simulink model "sogi_pll"  (R2023b)
settings: Solver=VariableStepAuto  StartTime=0.0  StopTime=50e-2  RelTol=1e-3
libraries: spsAlphaBetaZerotodq0Lib x2
settings Model: Creator=sabar  LastModifiedBy=sabar

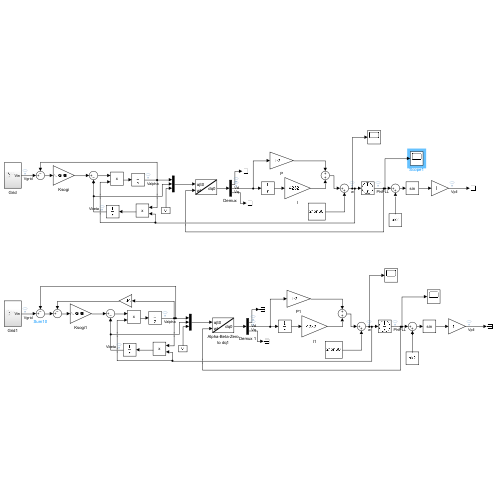
[thumbnail: Simulink's stored preview of the top-level diagram]
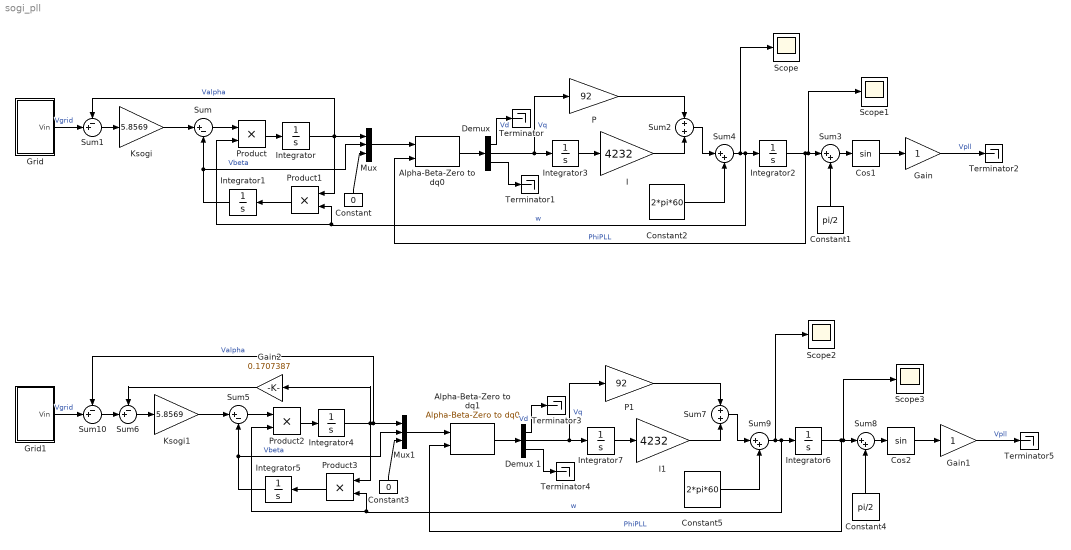
== system sogi_pll ==
  Alpha-Beta-Zero to dq0 : spsAlphaBetaZerotodq0Lib/Alpha-Beta-Zero to dq0  Alignment=Aligned with phase A axis
  Alpha-Beta-Zero to dq1 : spsAlphaBetaZerotodq0Lib/Alpha-Beta-Zero to dq0  Alignment=Aligned with phase A axis
  Constant : Constant  Value=0
  Constant1 : Constant  Value=pi/2
  Constant2 : Constant  Value=2*pi*60
  Constant3 : Constant  Value=0
  Constant4 : Constant  Value=pi/2
  Constant5 : Constant  Value=2*pi*60
  Cos1 : Trigonometry
  Cos2 : Trigonometry
  "Demux " : Demux  Outputs=3
  Demux 1 : Demux  Outputs=3
  Gain : Gain
  Gain1 : Gain
  Gain2 : Gain  Gain=0.1707387
  Grid : Subsystem
  Grid1 : Subsystem
  I : Gain  Gain=4232
  I1 : Gain  Gain=4232
  Integrator{,1,4..5} (4 alike) : Integrator  UpperSaturationLimit=1e3  LowerSaturationLimit=-1e3
  Integrator2 : Integrator  WrapState=on
  Integrator3 : Integrator
  Integrator6 : Integrator  WrapState=on
  Integrator7 : Integrator
  Ksogi : Gain  Gain=5.8569
  Ksogi1 : Gain  Gain=5.8569
  Mux : Mux  Inputs=3
  Mux1 : Mux  Inputs=3
  P : Gain  Gain=92
  P1 : Gain  Gain=92
  Product{,1..3} (4 alike) : Product
  Scope{,1..3} (4 alike) : Scope
  Sum : Sum  Inputs=|+-
  Sum1 : Sum  Inputs=-+|
  Sum10 : Sum  Inputs=-+|
  Sum2 : Sum  Inputs=+|+
  Sum{3..4,8..9} (4 alike) : Sum  Inputs=|++
  Sum5 : Sum  Inputs=|+-
  Sum6 : Sum  Inputs=-+|
  Sum7 : Sum  Inputs=+|+
  Terminator{,1..5} (6 alike) : Terminator
  wires:
  Sum2/1 -> Sum4/1
  Sum4/1 -> Scope/1, Product/2, Product1/2, Integrator2/1  "w"
  Constant/1 -> Mux/3
  Constant1/1 -> Sum3/2
  Sum3/1 -> Cos1/1
  Integrator2/1 -> Scope1/1, Sum3/1, Alpha-Beta-Zero to dq0/2  "PhiPLL"
  Cos1/1 -> Gain/1
  Gain/1 -> Terminator2/1  "Vpll"
  I/1 -> Sum2/2
  P/1 -> Sum2/1
  "Demux "/2 -> P/1, Integrator3/1  "Vq"
  Integrator3/1 -> I/1
  Constant2/1 -> Sum4/2
  "Demux "/3 -> Terminator1/1
  Integrator1/1 -> Mux/2, Sum/2  "Vbeta"
  "Demux "/1 -> Terminator/1  "Vd"
  Mux/1 -> Alpha-Beta-Zero to dq0/1
  Alpha-Beta-Zero to dq0/1 -> "Demux "/1
  Sum/1 -> Product/1
  Grid/1(Vin) -> Sum1/2  "Vgrid"
  Sum1/1 -> Ksogi/1
  Ksogi/1 -> Sum/1
  Product1/1 -> Integrator1/1
  Integrator/1 -> Product1/1, Mux/1, Sum1/1  "Valpha"
  Product/1 -> Integrator/1
  Product2/1 -> Integrator4/1
  Mux1/1 -> Alpha-Beta-Zero to dq1/1
  Ksogi1/1 -> Sum5/1
  Product3/1 -> Integrator5/1
  Sum5/1 -> Product2/1
  Demux 1/1 -> Terminator3/1  "Vd"
  Alpha-Beta-Zero to dq1/1 -> Demux 1/1
  Demux 1/3 -> Terminator4/1
  Constant5/1 -> Sum9/2
  P1/1 -> Sum7/1
  Cos2/1 -> Gain1/1
  Integrator7/1 -> I1/1
  Gain1/1 -> Terminator5/1  "Vpll"
  Integrator6/1 -> Scope3/1, Sum8/1, Alpha-Beta-Zero to dq1/2  "PhiPLL"
  Demux 1/2 -> P1/1, Integrator7/1  "Vq"
  I1/1 -> Sum7/2
  Sum7/1 -> Sum9/1
  Sum8/1 -> Cos2/1
  Integrator5/1 -> Mux1/2, Sum5/2  "Vbeta"
  Constant4/1 -> Sum8/2
  Constant3/1 -> Mux1/3
  Sum9/1 -> Scope2/1, Product2/2, Product3/2, Integrator6/1  "w"
  Sum6/1 -> Ksogi1/1
  Integrator4/1 -> Product3/1, Mux1/1, Sum10/1, Gain2/1  "Valpha"
  Gain2/1 -> Sum6/1
  Sum10/1 -> Sum6/2
  Grid1/1(Vin) -> Sum10/2  "Vgrid"

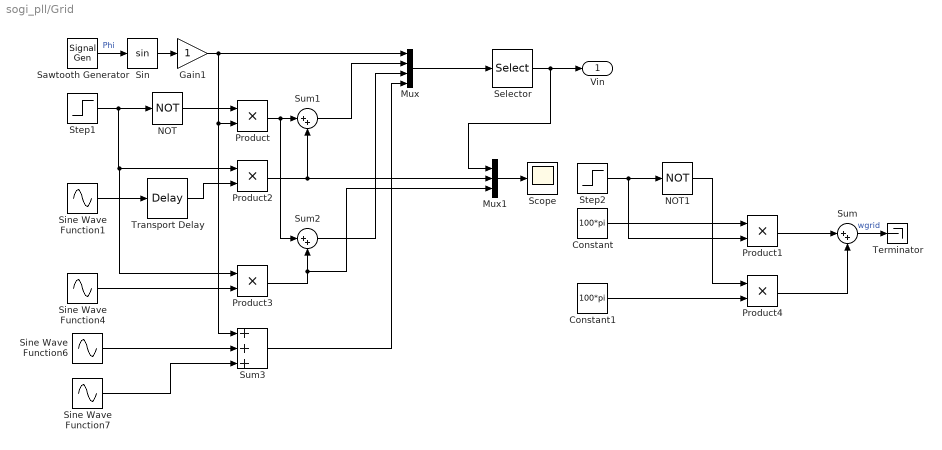
== system sogi_pll/Grid ==
  Constant : Constant  Value=100*pi
  Constant1 : Constant  Value=100*pi
  Gain1 : Gain
  Mux : Mux
  Mux1 : Mux  Inputs=3
  NOT : Logic  Operator=NOT  IconShape=distinctive  AllPortsSameDT=off  OutDataTypeStr=boolean
  NOT1 : Logic  Operator=NOT  IconShape=distinctive  AllPortsSameDT=off  OutDataTypeStr=boolean
  Product{,1..4} (5 alike) : Product
  Sawtooth Generator : SignalGenerator  WaveForm=sawtooth  Amplitude=pi  Frequency=314.159  Units=rad/sec
  Scope : Scope
  Selector : Selector  InputPortWidth=4  IndexOptions=Index vector (dialog)  Indices=1  OutputSizes=1
  Sin : Trigonometry
  Sine Wave Function1 : Sin  Frequency=314.159  SampleTime=0
  Sine Wave Function4 : Sin  Frequency=314.159  Phase=pi  SampleTime=0
  Sine Wave Function6 : Sin  Amplitude=1*0.1  Frequency=5*100*pi  SampleTime=0
  Sine Wave Function7 : Sin  Amplitude=1*0.05  Frequency=10*100*pi  SampleTime=0
  Step1 : Step  SampleTime=0
  Step2 : Step  Before=1  After=0  SampleTime=0
  Sum : Sum  Inputs=|++
  Sum1 : Sum  Inputs=|++
  Sum2 : Sum  Inputs=|++
  Sum3 : Sum  Inputs=+++
  Terminator : Terminator
  Transport Delay : TransportDelay  DelayTime=1000e-3
  Vin : Outport
  wires:
  Transport Delay/1 -> Product2/2
  Sine Wave Function7/1 -> Sum3/3
  Sum/1 -> Terminator/1  "wgrid"
  Sum3/1 -> Mux/4
  Constant/1 -> Product1/1
  Sine Wave Function1/1 -> Transport Delay/1
  Sin/1 -> Gain1/1
  Sum2/1 -> Mux/3
  Sawtooth Generator/1 -> Sin/1  "Phi"
  Product3/1 -> Mux1/3, Sum2/2
  Step2/1 -> Product1/2, NOT1/1
  Sine Wave Function4/1 -> Product3/2
  NOT1/1 -> Product4/1
  Sine Wave Function6/1 -> Sum3/2
  Mux/1 -> Selector/1
  Mux1/1 -> Scope/1
  NOT/1 -> Product/1
  Gain1/1 -> Sum3/1, Product/2, Mux/1
  Product2/1 -> Mux1/2, Sum1/2
  Product/1 -> Sum2/1, Sum1/1
  Step1/1 -> Product3/1, Product2/1, NOT/1
  Product1/1 -> Sum/1
  Sum1/1 -> Mux/2
  Selector/1 -> Mux1/1, Vin/1
  Product4/1 -> Sum/2
  Constant1/1 -> Product4/2

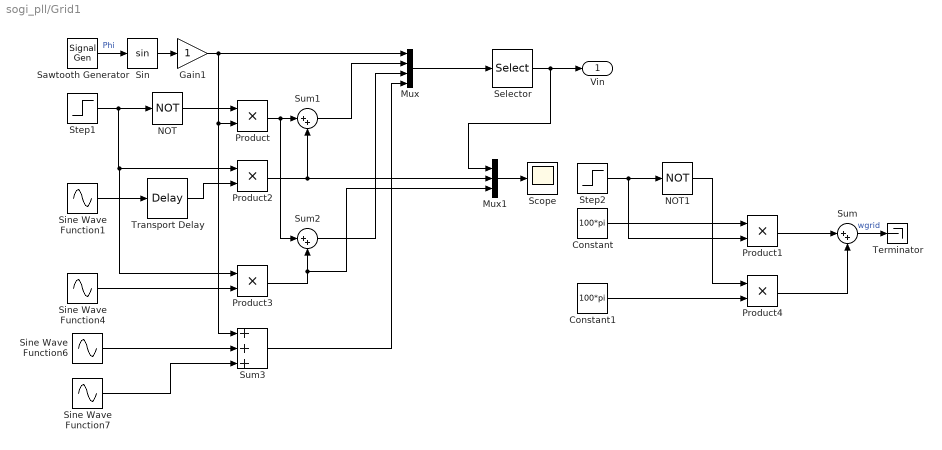
== system sogi_pll/Grid1 ==
  Constant : Constant  Value=100*pi
  Constant1 : Constant  Value=100*pi
  Gain1 : Gain
  Mux : Mux
  Mux1 : Mux  Inputs=3
  NOT : Logic  Operator=NOT  IconShape=distinctive  AllPortsSameDT=off  OutDataTypeStr=boolean
  NOT1 : Logic  Operator=NOT  IconShape=distinctive  AllPortsSameDT=off  OutDataTypeStr=boolean
  Product{,1..4} (5 alike) : Product
  Sawtooth Generator : SignalGenerator  WaveForm=sawtooth  Amplitude=pi  Frequency=314.159  Units=rad/sec
  Scope : Scope
  Selector : Selector  InputPortWidth=4  IndexOptions=Index vector (dialog)  Indices=1  OutputSizes=1
  Sin : Trigonometry
  Sine Wave Function1 : Sin  Frequency=314.159  SampleTime=0
  Sine Wave Function4 : Sin  Frequency=314.159  Phase=pi  SampleTime=0
  Sine Wave Function6 : Sin  Amplitude=1*0.1  Frequency=5*100*pi  SampleTime=0
  Sine Wave Function7 : Sin  Amplitude=1*0.05  Frequency=10*100*pi  SampleTime=0
  Step1 : Step  SampleTime=0
  Step2 : Step  Before=1  After=0  SampleTime=0
  Sum : Sum  Inputs=|++
  Sum1 : Sum  Inputs=|++
  Sum2 : Sum  Inputs=|++
  Sum3 : Sum  Inputs=+++
  Terminator : Terminator
  Transport Delay : TransportDelay  DelayTime=1000e-3
  Vin : Outport
  wires:
  Transport Delay/1 -> Product2/2
  Sine Wave Function7/1 -> Sum3/3
  Sum/1 -> Terminator/1  "wgrid"
  Sum3/1 -> Mux/4
  Constant/1 -> Product1/1
  Sine Wave Function1/1 -> Transport Delay/1
  Sin/1 -> Gain1/1
  Sum2/1 -> Mux/3
  Sawtooth Generator/1 -> Sin/1  "Phi"
  Product3/1 -> Mux1/3, Sum2/2
  Step2/1 -> Product1/2, NOT1/1
  Sine Wave Function4/1 -> Product3/2
  NOT1/1 -> Product4/1
  Sine Wave Function6/1 -> Sum3/2
  Mux/1 -> Selector/1
  Mux1/1 -> Scope/1
  NOT/1 -> Product/1
  Gain1/1 -> Sum3/1, Product/2, Mux/1
  Product2/1 -> Mux1/2, Sum1/2
  Product/1 -> Sum2/1, Sum1/1
  Step1/1 -> Product3/1, Product2/1, NOT/1
  Product1/1 -> Sum/1
  Sum1/1 -> Mux/2
  Selector/1 -> Mux1/1, Vin/1
  Product4/1 -> Sum/2
  Constant1/1 -> Product4/2
